simulink model "W2Q1"  (R2020b)
settings: Solver=VariableStepAuto  StartTime=0.0  StopTime=10.0  RelTol=1e-3
settings Model: Creator=VIVEK  LastModifiedBy=VIVEK

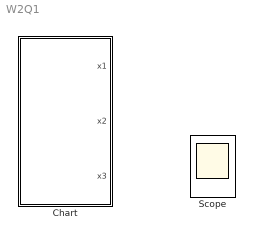
== system W2Q1 ==
  Chart : Stateflow chart  TreatAsAtomicUnit=on
  Scope : Scope  NumInputPorts=3
  wires:
  ? -> Scope/3
  ? -> Scope/2
  ? -> Scope/1

== stateflow chart W2Q1/Chart ==
  state State1
    entry:
    x2=0;
    x2=0;
    x1=0;
  state State2
    entry:
    x3=0;
    x2=0;
    x1=1;
  state State3
    entry:
    x3=0;
    x2=1;
    x1=0;
  state State4
    entry:
    x3=0;
    x2=1;
    x1=1;
  state State5
    entry:
    x3=1;
    x2=0;
    x1=0;
  (default) -> State1
  State5 -> State1 : {x1==1&&x2==0&&x3==0}
  State1 -> State2 : {x1==0&&x2==0&&x3==0}
  State2 -> State3 : {x1==0&&x2==0&&x3==1}
  State3 -> State4 : {x1==0&&x2==1&&x3==0}
  State4 -> State5 : {x1==0&&x2==1&&x3==1}
  data: x1 output; x2 output; x3 output
